simulink subsystem "PvtSubSys_VSM_SetSpd"  (R2020b)
settings: Solver=VariableStepAuto  StartTime=0.0  StopTime=10.0  RelTol=1e-3
undefined symbols (not defined in the file): ACC_STATE, P_VSM_PassSBRSpdIPLimt, P_VSM_TimeGapHMI_SW
libraries: simulink x6
settings Model: Creator=GW00133806  LastModifiedBy=GW00201299

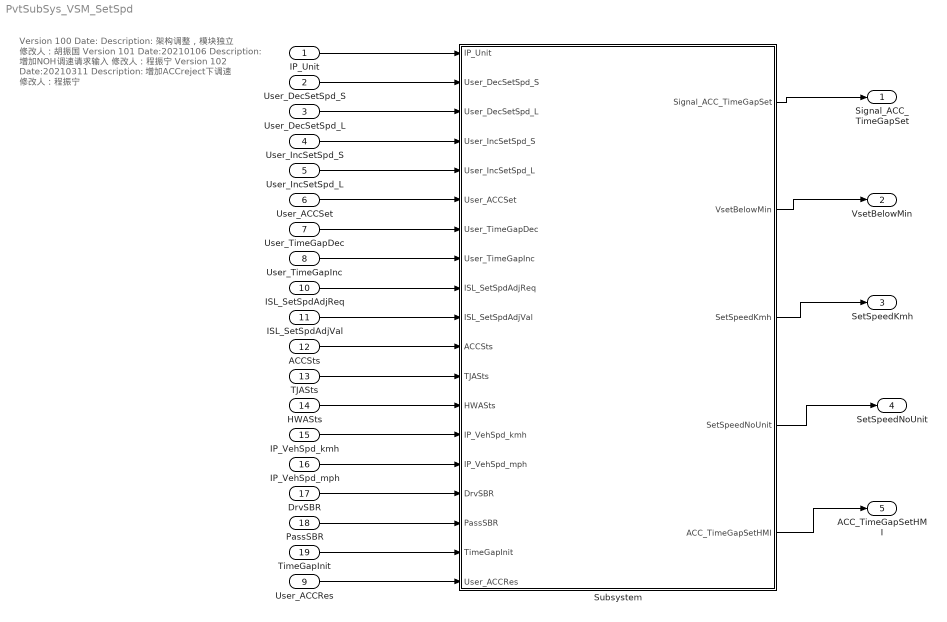
== system PvtSubSys_VSM_SetSpd ==
  note: Version 100
      | Date:
      | Description: 架构调整，模块独立
      | 修改人：胡振国
      | Version 101
      | Date:20210106
      | Description: 增加NOH调速请求输入
      | 修改人：程振宁
      | Version 102
      | Date:20210311
      | Description: 增加ACCreject下调速
      | 修改人：程振宁
  IP_Unit : Inport  OutDataTypeStr=boolean
  User_DecSetSpd_S : Inport  Port=2  OutDataTypeStr=boolean
  User_DecSetSpd_L : Inport  Port=3  OutDataTypeStr=boolean
  User_IncSetSpd_S : Inport  Port=4  OutDataTypeStr=boolean
  User_IncSetSpd_L : Inport  Port=5  OutDataTypeStr=boolean
  User_ACCSet : Inport  Port=6  OutDataTypeStr=boolean
  User_TimeGapDec : Inport  Port=7  OutDataTypeStr=boolean
  User_TimeGapInc : Inport  Port=8  OutDataTypeStr=boolean
  User_ACCRes : Inport  Port=9
  ISL_SetSpdAdjReq : Inport  Port=10  OutDataTypeStr=boolean
  ISL_SetSpdAdjVal : Inport  Port=11  OutDataTypeStr=uint8
  ACCSts : Inport  Port=12  OutDataTypeStr=Enum: ACC_STATE
  TJASts : Inport  Port=13  OutDataTypeStr=Enum: TJA_STATE
  HWASts : Inport  Port=14  OutDataTypeStr=Enum: HWA_STATE
  IP_VehSpd_kmh : Inport  Port=15  OutDataTypeStr=single
  IP_VehSpd_mph : Inport  Port=16  OutDataTypeStr=single
  DrvSBR : Inport  Port=17  OutDataTypeStr=boolean  LockScale=on
  PassSBR : Inport  Port=18  OutDataTypeStr=boolean
  TimeGapInit : Inport  Port=19
  Subsystem : Subsystem
  Signal_ACC_TimeGapSet : Outport  OutDataTypeStr=uint8
  VsetBelowMin : Outport  Port=2  OutDataTypeStr=boolean
  SetSpeedKmh : Outport  Port=3  OutDataTypeStr=single
  SetSpeedNoUnit : Outport  Port=4  OutDataTypeStr=uint8
  ACC_TimeGapSetHMI : Outport  Port=5
  wires:
  User_ACCRes/1 -> Subsystem/19(User_ACCRes)
  DrvSBR/1 -> Subsystem/16(DrvSBR)
  PassSBR/1 -> Subsystem/17(PassSBR)
  User_TimeGapDec/1 -> Subsystem/7(User_TimeGapDec)
  User_DecSetSpd_L/1 -> Subsystem/3(User_DecSetSpd_L)
  User_DecSetSpd_S/1 -> Subsystem/2(User_DecSetSpd_S)
  ACCSts/1 -> Subsystem/11(ACCSts)
  TJASts/1 -> Subsystem/12(TJASts)
  User_IncSetSpd_L/1 -> Subsystem/5(User_IncSetSpd_L)
  ISL_SetSpdAdjReq/1 -> Subsystem/9(ISL_SetSpdAdjReq)
  User_TimeGapInc/1 -> Subsystem/8(User_TimeGapInc)
  IP_VehSpd_kmh/1 -> Subsystem/14(IP_VehSpd_kmh)
  User_IncSetSpd_S/1 -> Subsystem/4(User_IncSetSpd_S)
  IP_VehSpd_mph/1 -> Subsystem/15(IP_VehSpd_mph)
  Subsystem/1(Signal_ACC_TimeGapSet) -> Signal_ACC_TimeGapSet/1
  User_ACCSet/1 -> Subsystem/6(User_ACCSet)
  IP_Unit/1 -> Subsystem/1(IP_Unit)
  ISL_SetSpdAdjVal/1 -> Subsystem/10(ISL_SetSpdAdjVal)
  HWASts/1 -> Subsystem/13(HWASts)
  Subsystem/3(SetSpeedKmh) -> SetSpeedKmh/1
  Subsystem/2(VsetBelowMin) -> VsetBelowMin/1
  Subsystem/4(SetSpeedNoUnit) -> SetSpeedNoUnit/1
  TimeGapInit/1 -> Subsystem/18(TimeGapInit)
  Subsystem/5(ACC_TimeGapSetHMI) -> ACC_TimeGapSetHMI/1

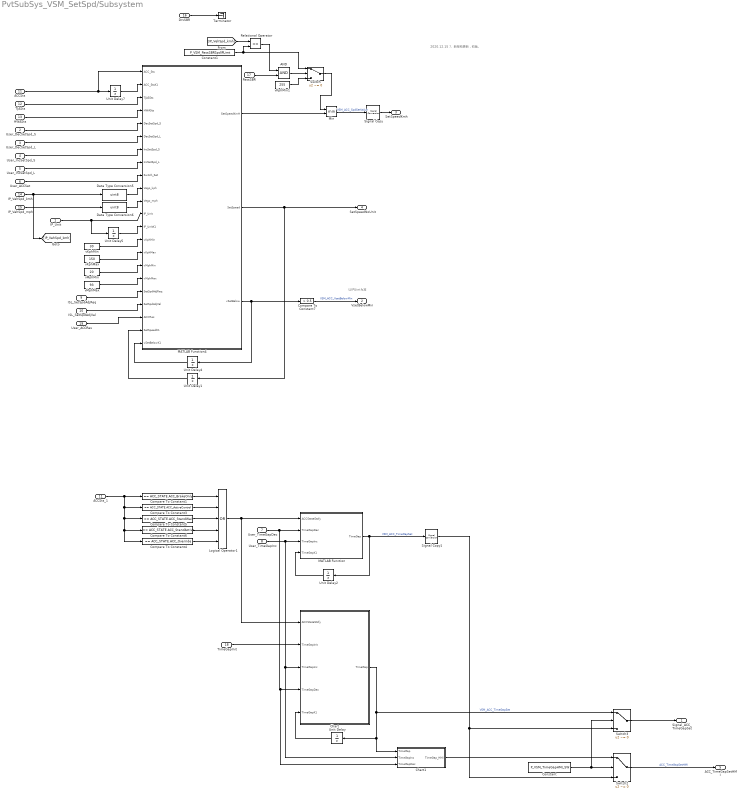
== system PvtSubSys_VSM_SetSpd/Subsystem ==
  note: 以IPUint为准
  note: 2020.12.15
      | 1、新架构更新，初版。
  IP_Unit : Inport  OutDataTypeStr=boolean
  User_DecSetSpd_S : Inport  Port=2  OutDataTypeStr=boolean
  User_DecSetSpd_L : Inport  Port=3  OutDataTypeStr=boolean
  User_IncSetSpd_S : Inport  Port=4  OutDataTypeStr=boolean
  User_IncSetSpd_L : Inport  Port=5  OutDataTypeStr=boolean
  User_ACCSet : Inport  Port=6  OutDataTypeStr=boolean
  User_TimeGapDec : Inport  Port=7  OutDataTypeStr=boolean
  User_TimeGapInc : Inport  Port=8  OutDataTypeStr=boolean
  ISL_SetSpdAdjReq : Inport  Port=9  OutDataTypeStr=boolean
  ISL_SetSpdAdjVal : Inport  Port=10  OutDataTypeStr=uint8
  ACCSts : Inport  Port=11  OutDataTypeStr=Enum: ACC_STATE
  TJASts : Inport  Port=12  OutDataTypeStr=Enum: TJA_STATE
  HWASts : Inport  Port=13  OutDataTypeStr=Enum: HWA_STATE
  IP_VehSpd_kmh : Inport  Port=14  OutDataTypeStr=single
  IP_VehSpd_mph : Inport  Port=15  OutDataTypeStr=single
  DrvSBR : Inport  Port=16  OutDataTypeStr=boolean  LockScale=on
  PassSBR : Inport  Port=17  OutDataTypeStr=boolean
  TimeGapInit : Inport  Port=18
  User_ACCRes : Inport  Port=19
  ACCSts_1 : InportShadow  Port=11  OutDataTypeStr=Enum: ACC_STATE
  AND : Logic  AllPortsSameDT=off  OutDataTypeStr=boolean
  Chart : Stateflow chart  TreatAsAtomicUnit=on
  Chart1 : Stateflow chart  TreatAsAtomicUnit=on
  Compare To Constant1 : simulink/Logic and Bit Operations/Compare To Constant  relop===  const=ACC_STATE.ACC_BrakeOnly  OutDataTypeStr=boolean
  Compare To Constant3 : simulink/Logic and Bit Operations/Compare To Constant  relop===  const=ACC_STATE.ACC_ActiveControl  OutDataTypeStr=boolean
  Compare To Constant4 : simulink/Logic and Bit Operations/Compare To Constant  relop===  const=ACC_STATE.ACC_Override  OutDataTypeStr=boolean
  Compare To Constant5 : simulink/Logic and Bit Operations/Compare To Constant  relop===  const=ACC_STATE.ACC_StandWait  OutDataTypeStr=boolean
  Compare To Constant6 : simulink/Logic and Bit Operations/Compare To Constant  relop===  const=ACC_STATE.ACC_StandActive  OutDataTypeStr=boolean
  Compare To Constant7 : simulink/Logic and Bit Operations/Compare To Constant  relop=>  const=0.5  OutDataTypeStr=boolean
  Constant : Constant  Value=P_VSM_TimeGapHMI_SW
  Constant1 : Constant  Value=P_VSM_PassSBRSpdIPLimt
  Data Type Conversion5 : DataTypeConversion  OutDataTypeStr=uint8
  Data Type Conversion6 : DataTypeConversion  OutDataTypeStr=uint8
  Logical Operator1 : Logic  Operator=OR  Inputs=5  AllPortsSameDT=off  OutDataTypeStr=boolean
  MATLAB Function : MATLAB Function  TreatAsAtomicUnit=on
  MATLAB Function4 : MATLAB Function  TreatAsAtomicUnit=on
  Min : MinMax  Inputs=2
  Relational Operator : RelationalOperator  Operator=<=  OutDataTypeStr=boolean  RndMeth=Simplest
  Signal Copy : SignalConversion  OverrideOpt=off
  Signal Copy1 : SignalConversion  OverrideOpt=off
  Switch : Switch  Criteria=u2 ~= 0
  Switch2 : Switch  Criteria=u2 ~= 0
  Switch3 : Switch  Criteria=u2 ~= 0
  Terminator : Terminator
  Unit Delay{,1,4..5} (4 alike) : UnitDelay  SampleTime=-1  HasFrameUpgradeWarning=on
  Unit Delay2 : UnitDelay  InitialCondition=4  SampleTime=-1  HasFrameUpgradeWarning=on
  Unit Delay7 : UnitDelay  InitialCondition=ACC_STATE.ACC_Off  SampleTime=-1  HasFrameUpgradeWarning=on
  vKphMax : Constant  Value=150  OutDataTypeStr=uint8
  vKphMin : Constant  Value=30  OutDataTypeStr=uint8
  vKphMin1 : Constant  Value=255  OutDataTypeStr=uint8
  vMphMax : Constant  Value=93  OutDataTypeStr=uint8
  vMphMin : Constant  Value=20  OutDataTypeStr=uint8
  Signal_ACC_TimeGapSet : Outport  OutDataTypeStr=uint8
  VsetBelowMin : Outport  Port=2  OutDataTypeStr=boolean
  SetSpeedKmh : Outport  Port=3  OutDataTypeStr=single
  SetSpeedNoUnit : Outport  Port=4  OutDataTypeStr=uint8
  ACC_TimeGapSetHMI : Outport  Port=5
  wires:
  Switch3/1 -> Signal_ACC_TimeGapSet/1
  Constant/1 -> Switch2/2, Switch3/2
  Signal Copy1/1 -> Switch2/3, Switch3/3
  Switch2/1 -> ACC_TimeGapSetHMI/1  "ACC_TimeGapSetHMI"
  TimeGapInit/1 -> Chart/2(TimeGapInit)
  Chart1/1(TimeGap_HMI) -> Switch2/1
  Unit Delay/1 -> Chart/5(TimeGapK1)
  Chart/1(TimeGap) -> Chart1/1(TimeGap), Unit Delay/1, Switch3/1  "VSM_ACC_TimeGapSet"
  User_TimeGapDec/1 -> MATLAB Function/2(TimeGapDec), Chart/4(TimeGapDec), Chart1/3(TimeGapDec)
  User_TimeGapInc/1 -> MATLAB Function/3(TimeGapInc), Chart/3(TimeGapInc), Chart1/2(TimeGapInc)
  Min/1 -> Signal Copy/1  "VSM_ACC_SpdSetValue"
  Compare To Constant4/1 -> Logical Operator1/5
  IP_VehSpd_kmh/1 -> [IP_VehSpd_kmh], Data Type Conversion5/1
  Compare To Constant5/1 -> Logical Operator1/3
  vKphMin/1 -> MATLAB Function4/14(vKphMin)
  Compare To Constant7/1 -> VsetBelowMin/1  "VSM_ACC_VsetBelowMin"
  User_DecSetSpd_L/1 -> MATLAB Function4/6(DecSetSpd_L)
  Compare To Constant3/1 -> Logical Operator1/2
  vMphMax/1 -> MATLAB Function4/17(vMphMax)
  vKphMax/1 -> MATLAB Function4/15(vKphMax)
  ACCSts/1 -> MATLAB Function4/1(ACC_Sts), Unit Delay7/1
  User_ACCSet/1 -> MATLAB Function4/9(Switch_Set)
  HWASts/1 -> MATLAB Function4/4(HWASts)
  vMphMin/1 -> MATLAB Function4/16(vMphMin)
  ISL_SetSpdAdjVal/1 -> MATLAB Function4/19(SetSpdAdjVal)
  Unit Delay2/1 -> MATLAB Function/4(TimeGapK1)
  Logical Operator1/1 -> MATLAB Function/1(ACCStateStsfy), Chart/1(ACCStateStsfy)
  Compare To Constant6/1 -> Logical Operator1/4
  MATLAB Function4/2(SetSpeed) -> Unit Delay1/1, SetSpeedNoUnit/1
  Data Type Conversion5/1 -> MATLAB Function4/10(Vego_kph)
  Unit Delay5/1 -> MATLAB Function4/13(IP_UnitK1)
  Data Type Conversion6/1 -> MATLAB Function4/11(Vego_mph)
  User_DecSetSpd_S/1 -> MATLAB Function4/5(DecSetSpd_S)
  MATLAB Function/1(TimeGap) -> Unit Delay2/1, Signal Copy1/1  "VSM_ACC_TimeGapSet"
  IP_Unit/1 -> Unit Delay5/1, MATLAB Function4/12(IP_Unit)
  User_IncSetSpd_L/1 -> MATLAB Function4/8(IncSetSpd_L)
  TJASts/1 -> MATLAB Function4/3(TJASSts)
  User_IncSetSpd_S/1 -> MATLAB Function4/7(IncSetSpd_S)
  Compare To Constant1/1 -> Logical Operator1/1
  MATLAB Function4/3(vSetBelow) -> Unit Delay4/1, Compare To Constant7/1
  IP_VehSpd_mph/1 -> Data Type Conversion6/1
  Unit Delay7/1 -> MATLAB Function4/2(ACC_StsK1)
  Unit Delay4/1 -> MATLAB Function4/22(vSetBelowK1)
  Signal Copy/1 -> SetSpeedKmh/1
  ACCSts_1/1 -> Compare To Constant3/1, Compare To Constant5/1, Compare To Constant6/1, Compare To Constant4/1, Compare To Constant1/1
  Unit Delay1/1 -> MATLAB Function4/21(SetSpeedK1)
  ISL_SetSpdAdjReq/1 -> MATLAB Function4/18(SetSpdAdjReq)
  PassSBR/1 -> AND/2
  DrvSBR/1 -> Terminator/1
  MATLAB Function4/1(SetSpeedKmH) -> Min/2
  Switch/1 -> Min/1
  [IP_VehSpd_kmh] -> Relational Operator/1
  AND/1 -> Switch/2
  Relational Operator/1 -> AND/1
  Constant1/1 -> Switch/1, Relational Operator/2
  vKphMin1/1 -> Switch/3
  User_ACCRes/1 -> MATLAB Function4/20(ACCRes)

== matlab function PvtSubSys_VSM_SetSpd/Subsystem/MATLAB Function4 ==
  data: SetSpeedKmH output; SetSpeed output uint8; ACC_Sts input Enum: ACC_STATE; ACC_StsK1 input Enum: ACC_STATE; TJASSts input; HWASts input; DecSetSpd_S input; DecSetSpd_L input; IncSetSpd_S input; IncSetSpd_L input; Switch_Set input; Vego_kph input; Vego_mph input; IP_Unit input; IP_UnitK1 input; vKphMin input; vKphMax input; vMphMin input; vMphMax input; SetSpdAdjReq input; SetSpdAdjVal input; ACCRes input; SetSpeedK1 input; vSetBelowK1 input; vSetBelow output
function [SetSpeedKmH,SetSpeed,vSetBelow] = ...
    TextInfo(ACC_Sts,ACC_StsK1,TJASSts,HWASts,DecSetSpd_S,DecSetSpd_L,IncSetSpd_S,IncSetSpd_L,Switch_Set,Vego_kph,Vego_mph,...
    IP_Unit,IP_UnitK1,...
    vKphMin,vKphMax,vMphMin,vMphMax,SetSpdAdjReq,SetSpdAdjVal,ACCRes, SetSpeedK1,vSetBelowK1)

SetSpeed = SetSpeedK1;
vSetBelow = max(0,vSetBelowK1 - 1);

if (ACC_Sts==ACC_STATE.ACC_ActiveControl||...
        ACC_Sts==ACC_STATE.ACC_Override||...
        ACC_Sts==ACC_STATE.ACC_StandActive)&&...
        (ACC_StsK1==ACC_STATE.ACC_Standby)&&...
        (TJASSts~=TJA_STATE.TJA_SafeStop || HWASts~=HWA_STATE.HWA_SafeStop)&&...
        (Switch_Set==true||ACCRes)                                           % 设置当前仪表车速用Switch_Set统一接口
    if IP_Unit==0
        SetSpeed = max(vKphMin,min(Vego_kph,vKphMax));        %  High Speed 150kph;
        vSetBelow = 10*(Vego_kph<vKphMin);
    else
        SetSpeed = max(vMphMin,min(Vego_mph,vMphMax));
        vSetBelow = 10*(Vego_mph<vMphMin);
    end
end

if ACCRes==true...
        &&(ACC_Sts==ACC_STATE.ACC_ActiveControl||ACC_Sts==ACC_STATE.ACC_Override||ACC_Sts==ACC_STATE.ACC_StandActive)...
        &&(ACC_StsK1==ACC_STATE.ACC_Standby)...
        &&(TJASSts~=TJA_STATE.TJA_SafeStop)
    if IP_Unit==0
        SetSpeed = SetSpeedK1;%  High Speed 150kph;
        vSetBelow = 10*(Vego_kph<vKphMin);
    else
        SetSpeed = SetSpeedK1;
        vSetBelow = 10*(Vego_mph<vMphMin);
    end   
end

% override时set当前车速为巡航车速
if Switch_Set==true...
        &&(ACC_Sts==ACC_STATE.ACC_Override && ACC_StsK1==ACC_STATE.ACC_Override && TJASSts~=TJA_STATE.TJA_SafeStop)...
        &&((IP_Unit==0 && SetSpeed < Vego_kph) || (IP_Unit~=0 && SetSpeed < Vego_mph))
    if IP_Unit==0
        SetSpeed = max(vKphMin,min(Vego_kph,vKphMax));%  High Speed 150kph;
        vSetBelow = 10*(Vego_kph<vKphMin);
    else
        SetSpeed = max(vMphMin,min(Vego_mph,vMphMax));
        vSetBelow = 10*(Vego_mph<vMphMin);
    end   
end

%可调速条件
if (...
   (ACC_Sts==ACC_STATE.ACC_ActiveControl && ACC_StsK1==ACC_STATE.ACC_ActiveControl)...
   ||(ACC_Sts==ACC_STATE.ACC_StandWait && ACC_StsK1==ACC_STATE.ACC_StandWait)...
   ||(ACC_Sts==ACC_STATE.ACC_StandActive && ACC_StsK1==ACC_STATE.ACC_StandActive)...
    )...
    &&(TJASSts~=TJA_STATE.TJA_SafeStop || HWASts~=HWA_STATE.HWA_SafeStop)
   
    if IP_Unit==0
        if DecSetSpd_S==true
            if mod(SetSpeedK1,5)==0
                if SetSpeedK1==vKphMin
                    vSetBelow = 10;
                else
                    SetSpeed = SetSpeedK1 - 5;
                end
            else
                SetSpeed = SetSpeedK1 - mod(SetSpeedK1,5);
            end
        end
        if DecSetSpd_L==true
            if mod(SetSpeedK1,5)==0
                if SetSpeedK1==vKphMin
                    vSetBelow = 10;
                else
                    SetSpeed = SetSpeedK1 - 10;
                end
            else
                SetSpeed = SetSpeedK1 - mod(SetSpeedK1,5);
            end
        end
        if IncSetSpd_S==true
            if mod(SetSpeedK1,5)==0
                SetSpeed = min(SetSpeedK1 + 5,vKphMax);
            else
                SetSpeed = SetSpeedK1 - mod(SetSpeedK1,5) + 5;
            end
        end
        if IncSetSpd_L==true
            if mod(SetSpeedK1,5)==0
                SetSpeed = min(SetSpeedK1 + 10,vKphMax);
            else
                SetSpeed = SetSpeedK1 - mod(SetSpeedK1,5) + 5;
            end
        end
        SetSpeed = max(vKphMin,min(vKphMax,SetSpeed));
    else
        if DecSetSpd_S==true
            if SetSpeedK1==vMphMin
                vSetBelow = 10;
            else
                SetSpeed = SetSpeedK1 - 1;
            end
        end
        if DecSetSpd_L==true
            if mod(SetSpeedK1,5)==0
                if SetSpeedK1==vMphMin
                    vSetBelow = 10;
                else
                    SetSpeed = SetSpeedK1 - 5;
                end
            else
                SetSpeed = SetSpeedK1 - mod(SetSpeedK1,5);
            end
        end
        if IncSetSpd_S==true
            SetSpeed = min(SetSpeedK1 + 5,vMphMax);
        end
        if IncSetSpd_L==true
            if mod(SetSpeedK1,5)==0
                SetSpeed = min(SetSpeedK1 + 5,vMphMax);
            else
                SetSpeed = SetSpeedK1 - mod(SetSpeedK1,5) + 5;
            end
        end
        SetSpeed = max(vMphMin,min(vMphMax,SetSpeed));
    end
end

% if (ACC_Sts==ACC_STATE.ACC_Override)&&...
%         (ACC_StsK1==ACC_STATE.ACC_Override)&&...
%         (SetS==true||SetL==true)
%     if IP_Unit==0
%         SetSpeed = max(vKphMin,min(Vego_kph,vKphMax));
%     else
%         SetSpeed = max(vMphMin,min(Vego_mph,vMphMax));
%     end
% end

% 新需求：Override可操作加速，不可操作减速，亦不可设置当前车速；
if (ACC_Sts==ACC_STATE.ACC_Override)&&...
        (ACC_StsK1==ACC_STATE.ACC_Override)&&...
        (TJASSts~=TJA_STATE.TJA_SafeStop || HWASts~=HWA_STATE.HWA_SafeStop)
    if IP_Unit==0
        if IncSetSpd_S==true
            if mod(SetSpeedK1,5)==0
                SetSpeed = min(SetSpeedK1 + 5,vKphMax);
            else
                SetSpeed = SetSpeedK1 - mod(SetSpeedK1,5) + 5;
            end
        end
        if IncSetSpd_L==true
            if mod(SetSpeedK1,5)==0
                SetSpeed = min(SetSpeedK1 + 10,vKphMax);
            else
                SetSpeed = SetSpeedK1 - mod(SetSpeedK1,5) + 5;
            end
        end
        SetSpeed = max(vKphMin,min(vKphMax,SetSpeed));
    else
        
        if IncSetSpd_S==true
            SetSpeed = min(SetSpeedK1 + 5,vMphMax);
        end
        if IncSetSpd_L==true
            if mod(SetSpeedK1,5)==0
                SetSpeed = min(SetSpeedK1 + 5,vMphMax);
            else
                SetSpeed = SetSpeedK1 - mod(SetSpeedK1,5) + 5;
            end
        end
        SetSpeed = max(vMphMin,min(vMphMax,SetSpeed));
    end
end


if (IP_UnitK1==0)&&(IP_Unit==1)
    if SetSpeed<255
        SetSpeed = max(min(round(SetSpeed*0.621),vMphMax),vMphMin);
    end
end
if (IP_UnitK1==1)&&(IP_Unit==0)
    if SetSpeed<255
        SetSpeed = max(min(round(SetSpeed*1.609),vKphMax),vKphMin);
    end
end


if SetSpdAdjReq %SetSpdAdjVal接口统一为公制单位。
    if IP_Unit==0
        SetSpeed = max(vKphMin,min(SetSpdAdjVal,vKphMax));%若当前仪表为公制单位则直接使用
    else
        SetSpeed = max(vMphMin,min(round(SetSpdAdjVal*0.62137),vMphMax));%若当前仪表为英制单位，取最接近的
    end
end

if IP_Unit==0
    SetSpeedKmH=single(SetSpeed);%公制单位的SetSpd输出
else
    SetSpeedKmH=single(SetSpeed*1.609);%公制单位的SetSpd输出
end

end

== stateflow chart PvtSubSys_VSM_SetSpd/Subsystem/Chart1 ==
  state Gapint
    en:
    TimeGap_HMI = 0;
  state Gap
    en:
    Cnt =uint8(0);
    TimeGap_HMI = TimeGap;
    du:
    TimeGap_HMI = TimeGap;
    Cnt = min(Cnt+uint8(1), uint8(150));
    if TimeGapInc==true ||TimeGapDec ==true
    Cnt = 0;
    end
  (default) -> Gapint
  Gapint -> Gap : [TimeGapInc == true||TimeGapDec  == true]
  Gap -> Gapint : [Cnt>149]
  data: TimeGap input; TimeGapInc input; TimeGapDec input; TimeGap_HMI output; Cnt local

== stateflow chart PvtSubSys_VSM_SetSpd/Subsystem/Chart ==
  state TimeGapinit
    TimeGap = TimeGapInit;
  state TimeGapSet
    TimeGapSet -> (junction 8)
    (junction 8) -> (junction 10) [order 1] : [ACCStateStsfy==true]
    (junction 10) -> (junction 15) [order 1] : [TimeGapDec==true]
    (junction 15) -> (junction 20) [order 2]
    (junction 8) -> (junction 31) [order 2]
    (junction 10) -> (junction 14) [order 2] : [TimeGapInc==true]
    (junction 15) -> (junction 18) [order 1] : [TimeGapK1==1]{TimeGap = uint8(1);}
    (junction 20) -> (junction 22) : {TimeGap = TimeGapK1 - uint8(1);}
    (junction 14) -> (junction 26) [order 2]
    (junction 14) -> (junction 24) [order 1] : [TimeGapK1==4]{TimeGap = uint8(4);}
    (junction 26) -> (junction 28) : {TimeGap = TimeGapK1 + uint8(1);}
    (junction 24) -> (junction 31)
    (junction 28) -> (junction 24)
    (junction 18) -> (junction 28)
    (junction 22) -> (junction 18)
  (default) -> TimeGapinit
  TimeGapinit -> TimeGapSet
  data: ACCStateStsfy input boolean; TimeGapInit input uint8; TimeGapInc input boolean; TimeGapDec input boolean; TimeGapK1 input uint8; TimeGap output uint8

== matlab function PvtSubSys_VSM_SetSpd/Subsystem/MATLAB Function ==
  data: ACCStateStsfy input; TimeGapDec input; TimeGapInc input; TimeGapK1 input uint8; TimeGap output uint8
function TimeGap= GapCalc(ACCStateStsfy,TimeGapDec,TimeGapInc,TimeGapK1)
if ACCStateStsfy==true
    if TimeGapDec==true
        if TimeGapK1==1
            TimeGap = uint8(1);
        else
            TimeGap = TimeGapK1 - uint8(1);
        end
    elseif TimeGapInc==true
        if TimeGapK1==uint8(4)
            TimeGap = uint8(4);
        else
            TimeGap = TimeGapK1 + uint8(1);
        end
    else
        TimeGap = TimeGapK1;
    end
else
    TimeGap = TimeGapK1;
end
end
